simulink model "_LD_V2"  (R2019a)
settings: Solver=ode4  StartTime=0.0  StopTime=10.0  FixedStep=0.001  RelTol=1e-3
model workspace (MAT data in the model file):
  FBv = [-0.360628002737 -0.359628002737 -0.358628002737 -0.357628002737 -0.356628002737 -0.355628002737 -0.354628002737 -0.353628002737 -0.352628002737 -0.351628002737 -0.350628002737 -0.349628002737 ... (3119 elements, 1x3119)]
  G_g = 16.59
  G_h = 8.17
  g = 9.81
  h_s = 0.5
  l = 2.8
  l_v = 1.344
  reifenX = [0 0.25 1]
  reifenY = [0 1 1]
  useController = 1
  v0 = 22.2222222222
  z_time = [0 1.5 1.95 2.15 10]
  z_vals = [0 0 0.1 1 1]
  zh_z = 1
  zv_z = 1
libraries: simulink x3
(part 1 of 2)
settings Model: Creator=phlippe  LastModifiedBy=Mel
settings DataIOCC: ReturnWorkspaceOutputs=off
settings DebuggingCC: ArithmeticOperatorsInVariantConditions=warning
settings SFSimCC: SimUseLocalCustomCode=off
settings RTWCC: RTWUseLocalCustomCode=off

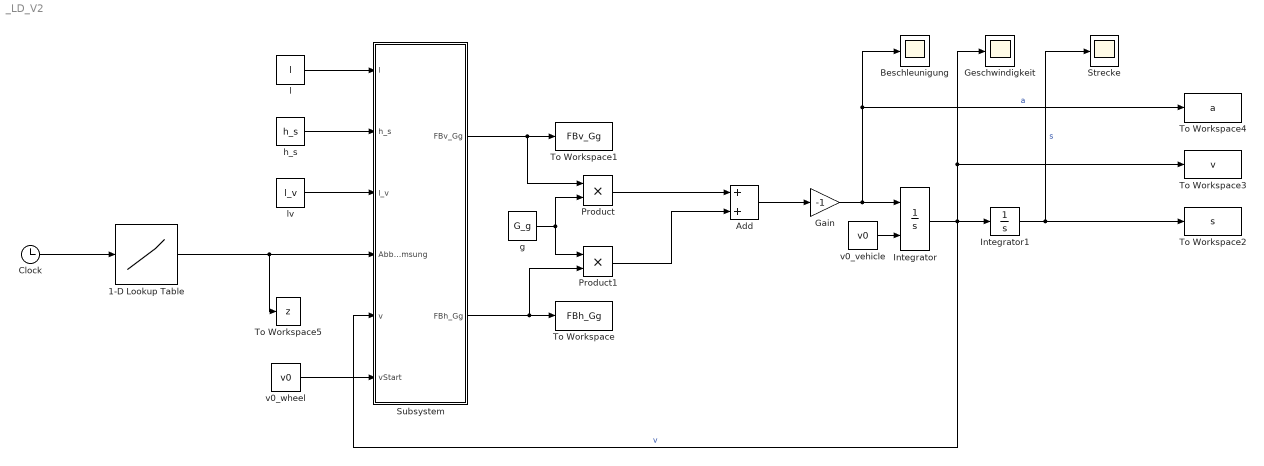
== system _LD_V2 ==
  1-D Lookup Table : Lookup_n-D  NumberOfTableDimensions=1  BreakpointsForDimension1=z_time  Table=z_vals  ExtrapMethod=Clip  UseLastTableValue=on  InternalRulePriority=Speed  RndMeth=Simplest  InputSameDT=on
  Add : Sum
  Beschleunigung : Scope
  Clock : Clock
  Gain : Gain  Gain=-1
  Geschwindigkeit : Scope
  Integrator : Integrator  InitialConditionSource=external  LimitOutput=on  LowerSaturationLimit=0
  Integrator1 : Integrator
  Product : Product
  Product1 : Product
  Strecke : Scope
  Subsystem : Subsystem
  To Workspace : ToWorkspace  VariableName=FBh_Gg  SaveFormat=Timeseries  SampleTime=-1
  To Workspace1 : ToWorkspace  VariableName=FBv_Gg  SaveFormat=Timeseries  SampleTime=-1
  To Workspace2 : ToWorkspace  VariableName=s  SaveFormat=Timeseries  SampleTime=-1
  To Workspace3 : ToWorkspace  VariableName=v  SaveFormat=Timeseries  SampleTime=-1
  To Workspace4 : ToWorkspace  VariableName=a  SaveFormat=Timeseries  SampleTime=-1
  To Workspace5 : ToWorkspace  VariableName=z  SaveFormat=Timeseries  SampleTime=-1
  "g " : Constant  Value=G_g
  h_s : Constant  Value=h_s
  l : Constant  Value=l
  "lv " : Constant  Value=l_v
  v0_vehicle : Constant  Value=v0
  v0_wheel : Constant  Value=v0
  wires:
  h_s/1 -> Subsystem/2(h_s)
  l/1 -> Subsystem/1(l)
  "lv "/1 -> Subsystem/3(l_v)
  1-D Lookup Table/1 -> To Workspace5/1, Subsystem/4(Abbremsung)
  Clock/1 -> 1-D Lookup Table/1
  Subsystem/1(FBv_Gg) -> Product/1, To Workspace1/1
  "g "/1 -> Product1/1, Product/2
  Product/1 -> Add/1
  Product1/1 -> Add/2
  Add/1 -> Gain/1
  v0_vehicle/1 -> Integrator/2
  Gain/1 -> Integrator/1, Beschleunigung/1, To Workspace4/1  "a"
  Integrator1/1 -> Strecke/1, To Workspace2/1  "s"
  Integrator/1 -> To Workspace3/1, Geschwindigkeit/1, Subsystem/5(v), Integrator1/1  "v"
  Subsystem/2(FBh_Gg) -> Product1/2, To Workspace/1
  v0_wheel/1 -> Subsystem/6(vStart)

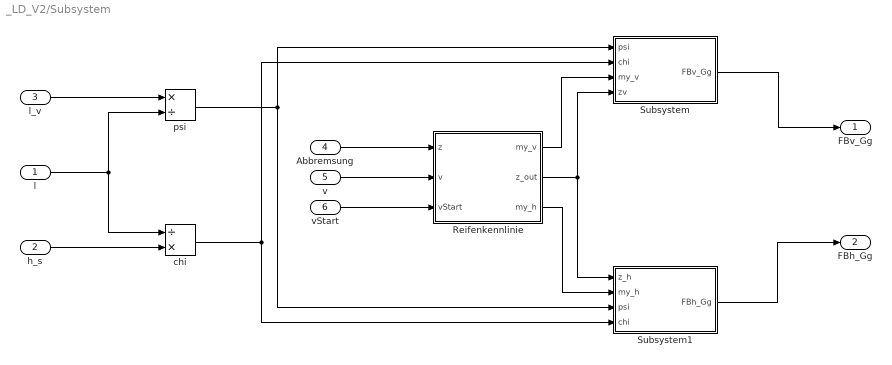
== system _LD_V2/Subsystem ==
  l : Inport
  h_s : Inport  Port=2
  l_v : Inport  Port=3
  Abbremsung : Inport  Port=4
  v : Inport  Port=5
  vStart : Inport  Port=6
  Reifenkennlinie : Subsystem
  Subsystem : Subsystem
  Subsystem1 : Subsystem
  chi : Product  Inputs=/*
  "psi " : Product  Inputs=*/
  FBv_Gg : Outport
  FBh_Gg : Outport  Port=2
  wires:
  h_s/1 -> chi/2
  l/1 -> chi/1, "psi "/2
  l_v/1 -> "psi "/1
  Subsystem/1(FBv_Gg) -> FBv_Gg/1
  "psi "/1 -> Subsystem/1(psi), Subsystem1/3(psi)
  chi/1 -> Subsystem1/4(chi), Subsystem/2(chi)
  Subsystem1/1(FBh_Gg) -> FBh_Gg/1
  v/1 -> Reifenkennlinie/2(v)
  Abbremsung/1 -> Reifenkennlinie/1(z)
  Reifenkennlinie/1(my_v) -> Subsystem/3(my_v)
  Reifenkennlinie/2(z_out) -> Subsystem1/1(z_h), Subsystem/4(zv)
  Reifenkennlinie/3(my_h) -> Subsystem1/2(my_h)
  vStart/1 -> Reifenkennlinie/3(vStart)

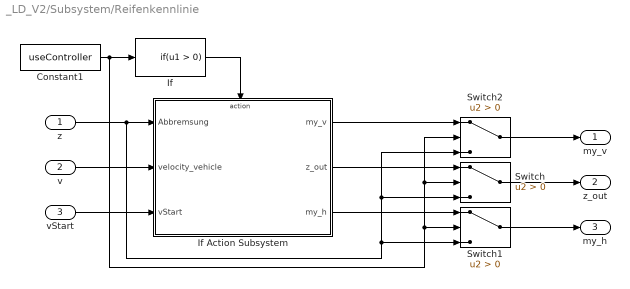
== system _LD_V2/Subsystem/Reifenkennlinie ==
  z : Inport
  v : Inport  Port=2
  vStart : Inport  Port=3
  Constant1 : Constant  Value=useController
  If : If  ShowElse=off
  If Action Subsystem : Subsystem  TreatAsAtomicUnit=on
  Switch : Switch  Criteria=u2 > Threshold
  Switch1 : Switch  Criteria=u2 > Threshold
  Switch2 : Switch  Criteria=u2 > Threshold
  my_v : Outport
  z_out : Outport  Port=2
  my_h : Outport  Port=3
  wires:
  z/1 -> Switch/3, Switch2/3, Switch1/3, If Action Subsystem/1(Abbremsung)
  v/1 -> If Action Subsystem/2(velocity_vehicle)
  vStart/1 -> If Action Subsystem/3(vStart)
  Constant1/1 -> Switch2/2, Switch/2, Switch1/2, If/1
  If Action Subsystem/2(z_out) -> Switch/1
  Switch/1 -> z_out/1
  Switch1/1 -> my_h/1
  If Action Subsystem/3(my_h) -> Switch1/1
  Switch2/1 -> my_v/1
  If Action Subsystem/1(my_v) -> Switch2/1
  If/1 -> If Action Subsystem/Action
